simulink model "IdealVS_R_3"  (R2014b)
settings: Solver=VariableStepAuto  StartTime=0.0  StopTime=0.3  RelTol=1e-3
libraries: fl_lib x14, nesl_utility x7
settings Model: Creator=mmi-vsa  LastModifiedBy=mmi-vsa
settings DataIOCC: LimitDataPoints=off  SaveFormat=Dataset
settings OptimizationCC: UseDivisionForNetSlopeComputation=off  LifeSpan=auto  SimCompilerOptimization=off
settings DebuggingCC: SolverPrmCheckMsg=none  FcnCallInpInsideContextMsg=error  FrameProcessingCompatibilityMsg=error  SFUnexpectedBacktrackingDiag=error  SFNoUnconditionalDefaultTransitionDiag=error
settings HardwareCC: ProdBitPerPointer=64  ProdLargestAtomicFloat=Float  ProdIntDivRoundTo=Zero  ProdEndianess=LittleEndian  ProdWordSize=64  ProdHWDeviceType=Intel->x86-64 (Windows64)
settings ModelReferenceCC: PropagateSignalLabelsOutOfModel=on
settings RTWCC: RTWCompilerOptimization=off
settings GRTTargetCC: TargetLangStandard=C99 (ISO)  GeneratePreprocessorConditionals=Use local settings

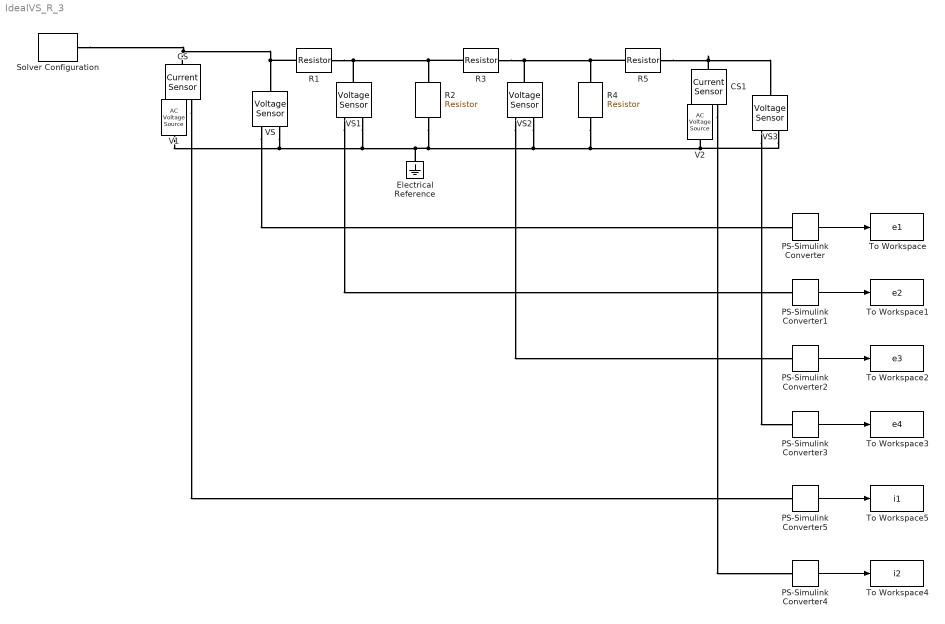
== system IdealVS_R_3 ==
  CS : fl_lib/Electrical/Electrical Sensors/Current Sensor
  CS1 : fl_lib/Electrical/Electrical Sensors/Current Sensor
  Electrical Reference : fl_lib/Electrical/Electrical Elements/Electrical Reference
  PS-Simulink Converter{,1..5} (6 alike) : nesl_utility/PS-Simulink Converter  PhysicalDomain=network_engine_domain  SubClassName=ps_output  LeftPortType=input  RightPortType=output  PseudoPeriodic=off  Frequencies=[]  Unit=1  AffineConversion=off
  R{1..5} (5 alike) : fl_lib/Electrical/Electrical Elements/Resistor  R=1 Ohm  i_specify=off  i_priority=High  i=0 A  v_specify=off  v_priority=High  v=0 V
  Solver Configuration : nesl_utility/Solver Configuration  PhysicalDomain=network_engine_domain  SubClassName=solver  LeftPortType=input  RightPortType=generic  Accelerate=off  Tones=[]  Harmonics=[]  SimulateNoise=off  Profile=off  UseLocalSampling=off  EnableSwitchedLinearOptims=on  FrequencyDomain=off  UseCCode=off  RelTol=0.001  AbsTol=1e-06  MinStep=1e-09  ToWorkspace=off  DoDC=off  ResidualTolerance=1e-09  UseLocalSolver=on  LocalSolverChoice=NE_TRAPEZOIDAL_ADVANCER  LocalSolverSampleTime=0.001  DoFixedCost=on  MaxNonlinIter=3  MaxModeIter=2  LinearAlgebra=Sparse  DelaysMemoryBudget=1024  AutomaticFiltering=on  FilteringTimeConstant=0.001
  To Workspace : ToWorkspace  VariableName=e1  SampleTime=-1
  To Workspace1 : ToWorkspace  VariableName=e2  SampleTime=-1
  To Workspace2 : ToWorkspace  VariableName=e3  SampleTime=-1
  To Workspace3 : ToWorkspace  VariableName=e4  SampleTime=-1
  To Workspace4 : ToWorkspace  VariableName=i2  SampleTime=-1
  To Workspace5 : ToWorkspace  VariableName=i1  SampleTime=-1
  V1 : fl_lib/Electrical/Electrical Sources/AC Voltage Source  amp=10 V  shift=90 deg  frequency=50 Hz  omega=0 rad/s
  V2 : fl_lib/Electrical/Electrical Sources/AC Voltage Source  amp=20 V  shift=90 deg  frequency=50 Hz  omega=0 rad/s
  VS{,1..3} (4 alike) : fl_lib/Electrical/Electrical Sensors/Voltage Sensor
  wires:
  PS-Simulink Converter/1 -> To Workspace/1
  PS-Simulink Converter1/1 -> To Workspace1/1
  PS-Simulink Converter2/1 -> To Workspace2/1
  PS-Simulink Converter3/1 -> To Workspace3/1
  PS-Simulink Converter4/1 -> To Workspace4/1
  PS-Simulink Converter5/1 -> To Workspace5/1
  connections:
  R1/LConn1 -- Solver Configuration/RConn1 -- CS/LConn1 -- VS/LConn1
  R1/RConn1 -- VS1/LConn1 -- R3/LConn1 -- R2/LConn1
  R3/RConn1 -- VS2/LConn1 -- R5/LConn1 -- R4/LConn1
  R5/RConn1 -- CS1/LConn1 -- VS3/LConn1
  VS2/RConn2 -- V1/RConn1 -- VS/RConn2 -- VS1/RConn2 -- Electrical Reference/LConn1 -- R2/RConn1 -- R4/RConn1 -- VS3/RConn2 -- V2/RConn1
  CS/RConn2 -- V1/LConn1
  VS/RConn1 -- PS-Simulink Converter/LConn1
  VS1/RConn1 -- PS-Simulink Converter1/LConn1
  VS2/RConn1 -- PS-Simulink Converter2/LConn1
  VS3/RConn1 -- PS-Simulink Converter3/LConn1
  CS1/RConn1 -- PS-Simulink Converter4/LConn1
  CS/RConn1 -- PS-Simulink Converter5/LConn1
  V2/LConn1 -- CS1/RConn2
